simulink model "a_MPC"  (R2021b)
settings: Solver=VariableStepAuto  StartTime=0.0  StopTime=15.0  RelTol=1e-3
values from neighbouring files (symbols this model uses):
  A = sysd.A    [main4.m]
  B = sysd.B    [main4.m]
  C = sysd.C    [main4.m]
  C_temp = eye(length(A))    [main4.m]
  D_temp = zeros(length(B), 1)    [main4.m]
  N1 = 5    [main4.m]
  N2 = 100    [main4.m]
  Q_LQ_3 = 0.1*eye(2)    [main4.m]
  QMPC1 = Q_LQ_1    [main4.m]
  QMPC2 = Q_LQ_1    [main4.m]
  R1 = R_LQ_1    (= 1)    [main4.m]
  R2 = R_LQ_1    (= 1)    [main4.m]
  R_LQ_3 = 1    [main4.m]
  S1 = Pr1    [main4.m]
  S2 = Pr1    [main4.m]
  S3 = Q_LQ_1    [main4.m]
  Ts = 0.1    [main4.m]
  u_max = 5    [main4.m]
  u_min = -5    [main4.m]
  x_0 = [0 10]'    [main4.m]
  xref = [0 0]'    [main4.m]
undefined symbols (not defined in the file or in its folder): LQ_d_1, mympc, N, umax, umin
settings Model: Creator=PaoloA  LastModifiedBy=PaoloA

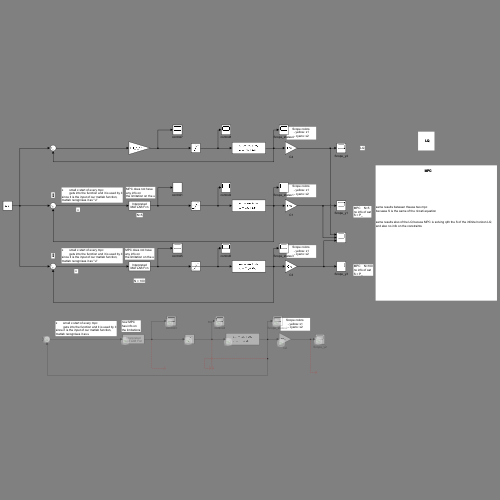
[thumbnail: Simulink's stored preview of the top-level diagram]
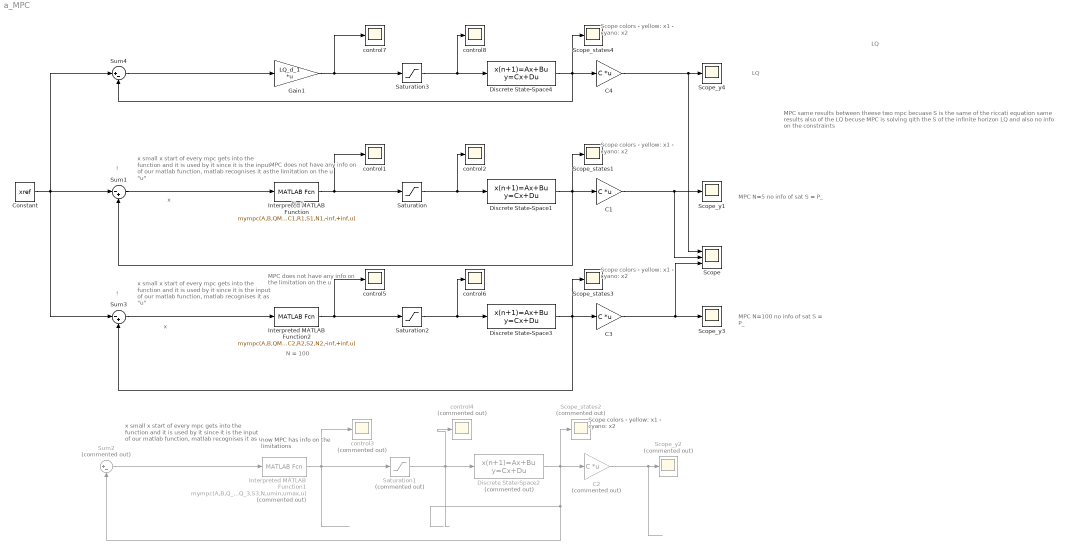
== system a_MPC ==
  note: LQ
  note: x
  note: !
  note: MPC    N=5
      | no info of sat
      | S = P_
  note: LQ
  note: MPC
      |
      | same results between theese two mpc
      | becuase S is the same of the riccati equation
      |
      | same results also of the LQ becuse MPC is solving qith the S of the infinite horizon LQ and also no info on the constraints
  note: N=5
  note: N = 100
  note: MPC does not have
      | any info on
      | the limitation on the u
  note: x       small x start of every mpc
      |          gets into the function and it is used by it
      | since it is the input of our matlab function,
      | matlab recognises it as "u"
  note: Scope colors
      | - yellow: x1
      | - cyano: x2
  note: x       small x start of every mpc
      |          gets into the function and it is used by it
      | since it is the input of our matlab function,
      | matlab recognises it as u
  note: Scope colors
      | - yellow: x1
      | - cyano: x2
  note: now MPC
      | has info on
      | the limitations
  note: x       small x start of every mpc
      |          gets into the function and it is used by it
      | since it is the input of our matlab function,
      | matlab recognises it as "u"
  note: Scope colors
      | - yellow: x1
      | - cyano: x2
  note: MPC does not have
      | any info on
      | the limitation on the u
  note: Scope colors
      | - yellow: x1
      | - cyano: x2
  note: MPC    N=100
      | no info of sat
      | S = P_
  note: !
  note: x
  C1 : Gain  Gain=C  Multiplication=Matrix(K*u)
  C2 : Gain  Commented=on  Gain=C  Multiplication=Matrix(K*u)
  C3 : Gain  Gain=C  Multiplication=Matrix(K*u)
  C4 : Gain  Gain=C  Multiplication=Matrix(K*u)
  Constant : Constant  Value=xref
  Discrete State-Space1 : DiscreteStateSpace  A=A  B=B  C=C_temp  D=D_temp  InitialCondition=x_0  SampleTime=Ts
  Discrete State-Space2 : DiscreteStateSpace  Commented=on  A=A  B=B  C=C_temp  D=D_temp  InitialCondition=x_0  SampleTime=Ts
  Discrete State-Space3 : DiscreteStateSpace  A=A  B=B  C=C_temp  D=D_temp  InitialCondition=x_0  SampleTime=Ts
  Discrete State-Space4 : DiscreteStateSpace  A=A  B=B  C=C_temp  D=D_temp  InitialCondition=x_0  SampleTime=Ts
  Gain1 : Gain  Gain=LQ_d_1  Multiplication=Matrix(K*u)
  Interpreted MATLAB Function : MATLABFcn  MATLABFcn=mympc(A,B,QMPC1,R1,S1,N1,-inf,+inf,u)  OutputDimensions=1
  Interpreted MATLAB Function1 : MATLABFcn  Commented=on  MATLABFcn=mympc(A,B,Q_LQ_3,R_LQ_3,S3,N,umin,umax,u)
  Interpreted MATLAB Function2 : MATLABFcn  MATLABFcn=mympc(A,B,QMPC2,R2,S2,N2,-inf,+inf,u)  OutputDimensions=1
  Saturation : Saturate  UpperLimit=u_max  LowerLimit=u_min
  Saturation1 : Saturate  Commented=on  UpperLimit=u_max  LowerLimit=u_min
  Saturation2 : Saturate  UpperLimit=u_max  LowerLimit=u_min
  Saturation3 : Saturate  UpperLimit=u_max  LowerLimit=u_min
  Scope : Scope  NumInputPorts=3
  Scope_states1 : Scope
  Scope_states2 : Scope  Commented=on
  Scope_states3 : Scope
  Scope_states4 : Scope
  Scope_y1 : Scope
  Scope_y2 : Scope  Commented=on
  Scope_y3 : Scope
  Scope_y4 : Scope
  Sum1 : Sum  Inputs=|-+
  Sum2 : Sum  Commented=on  Inputs=|+-
  Sum3 : Sum  Inputs=|-+
  Sum4 : Sum  Inputs=|+-
  control{1..2,5..8} (6 alike) : Scope
  control3 : Scope  Commented=on
  control4 : Scope  Commented=on
  wires:
  C1/1 -> Scope_y1/1, Scope/2
  Discrete State-Space1/1 -> C1/1, Scope_states1/1, Sum1/2
  Saturation/1 -> control2/1, Discrete State-Space1/1
  Sum1/1 -> Interpreted MATLAB Function/1
  Interpreted MATLAB Function/1 -> Saturation/1, control1/1
  Interpreted MATLAB Function1/1 -> Saturation1/1, control3/1
  Saturation1/1 -> control4/1, Discrete State-Space2/1
  C2/1 -> Scope_y2/1
  Discrete State-Space2/1 -> C2/1, Scope_states2/1, Sum2/2
  Sum2/1 -> Interpreted MATLAB Function1/1
  Interpreted MATLAB Function2/1 -> Saturation2/1, control5/1
  Saturation2/1 -> control6/1, Discrete State-Space3/1
  C3/1 -> Scope/3, Scope_y3/1
  Discrete State-Space3/1 -> C3/1, Scope_states3/1, Sum3/2
  Sum3/1 -> Interpreted MATLAB Function2/1
  Constant/1 -> Sum4/1, Sum3/1, Sum1/1
  C4/1 -> Scope/1, Scope_y4/1
  Saturation3/1 -> control8/1, Discrete State-Space4/1
  Discrete State-Space4/1 -> C4/1, Scope_states4/1, Sum4/2
  Sum4/1 -> Gain1/1
  Gain1/1 -> Saturation3/1, control7/1
